simulink model "DSHMwithHitting"  (R2013b)
settings: Solver=ode3  StartTime=0.0  StopTime=10.0  FixedStep=0.001  RelTol=1e-3
undefined symbols (not defined in the file): sigbuilder_block
libraries: simulink x1
settings Model: Creator=Deepak  LastModifiedBy=Deepak

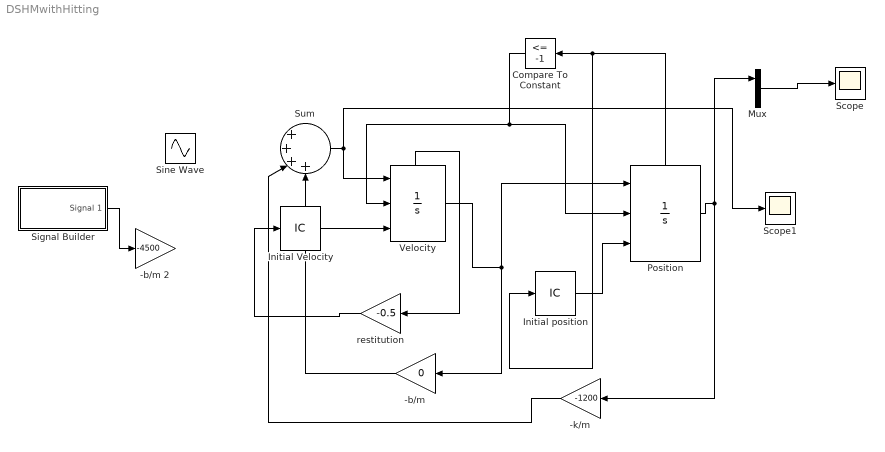
== system DSHMwithHitting ==
  "-b/m " : Gain  Gain=0
  -b/m 2 : Gain  Gain=-4500
  "-k/m " : Gain  Gain=-1200
  Compare To Constant : simulink/Logic and Bit Operations/Compare To Constant  relop=<=  const=-1  OutDataTypeStr=boolean
  "Initial Velocity " : InitialCondition  Value=0
  "Initial position " : InitialCondition  Value=4
  Mux : Mux  Inputs=2
  "Position " : Integrator  ExternalReset=rising  InitialConditionSource=external  LimitOutput=on  UpperSaturationLimit=200  LowerSaturationLimit=-2.0  ShowStatePort=on
  Scope : Scope
      settings: TimeRange=0.1287001287001287  YMin=-0.9436274509803924  YMax=0.1249999999999998
  Scope1 : Scope
  Signal Builder : Subsystem  Tag=STV Subsys  LoadFcn=sigbuilder_block('load');  StartFcn=sigbuilder_block('start');  StopFcn=sigbuilder_block('stop');  ClipboardFcn=sigbuilder_block('clipboard');  mask(Sigbuilder block){}
      mask help: Simulink:masks:SigbuilderBlock_MD
      mask init:
      | if ~strcmp(get_param(bdroot(gcbh),'SimulationStatus'),'stopped') tuvar = sigbuilder_block('maskInit'); end
      settings: CopyFcn=sigbuilder_block('copy');  DeleteFcn=sigbuilder_block('delete');  ModelCloseFcn=sigbuilder_block('modelClose');  PreSaveFcn=sigbuilder_block('preSave');  PauseFcn=sigbuilder_block('pause');  ContinueFcn=sigbuilder_block('continue');  NameChangeFcn=sigbuilder_block('namechange');  OpenFcn=sigbuilder_block('open',[436.656 202.84 549.567 399.685 ]);  CloseFcn=sigbuilder_block('close');
      mask Display: plot(0, 0, 100, 100,[2, 2, 32, 32, 2], [68, 8, 8, 68, 68],[32, 2], [38, 38], [32, 19, 2],[53, 60, 44], [32, 17, 17, 2],[16, 16, 31, 31]);txt = getActiveGroup(gcbh);text(2, 100, txt,'verticalAlignment', 'top');
  Sine Wave : Sin  Amplitude=1500  SampleTime=0
  Sum : Sum  Inputs=|++++
  "Velocity " : Integrator  ExternalReset=rising  InitialConditionSource=external  LimitOutput=on  UpperSaturationLimit=200  LowerSaturationLimit=-200  ShowStatePort=on
  "restitution " : Gain  Gain=-0.5
  wires:
  "Velocity "/1 -> "Position "/1, "-b/m "/1
  "Position "/1 -> "-k/m "/1, Mux/1
  "-b/m "/1 -> Sum/4
  Sum/1 -> Scope1/1, "Velocity "/1
  Mux/1 -> Scope/1
  "Initial Velocity "/1 -> "Velocity "/3
  "-k/m "/1 -> Sum/3
  Compare To Constant/1 -> "Velocity "/2, "Position "/2
  "Velocity "/State -> "restitution "/1
  "restitution "/1 -> "Initial Velocity "/1
  Signal Builder/1(Signal 1) -> -b/m 2/1
  "Initial position "/1 -> "Position "/3
  "Position "/State -> "Initial position "/1, Compare To Constant/1

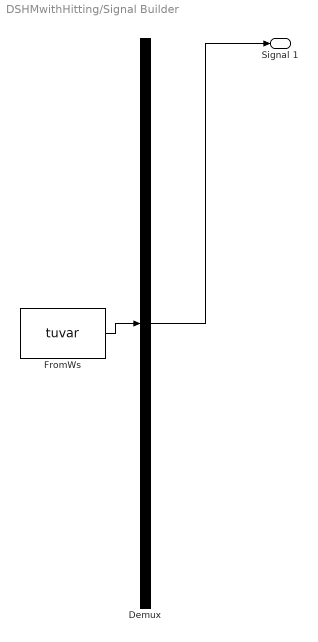
== system DSHMwithHitting/Signal Builder ==
  Demux : Demux  Tag=STV Demux  Outputs=1
  FromWs : FromWorkspace  Tag=STV FromWs  VariableName=tuvar  SampleTime=0
      SigBuilderData=|
      | common.afterFinalStr = 'Extrapolate'
      | common.sampleTime = 0
      | dataSet.timeRange = [0 10]
      | dataSet.name = 'Group 1'
      | sbobj.Groups.Name = 'Group 1'
      | sbobj.Groups.Signals.Name = 'Signal 1'
      | sbobj.Groups.Signals.XData = [0 4 4 4.3 4.3 10]
      | sbobj.Groups.Signals.YData = [0 0 2 2 0 0]
  Signal 1 : Outport  Tag=STV Outport
  wires:
  Demux/1 -> Signal 1/1
  FromWs/1 -> Demux/1
